simulink model "Torque_regulation_1_0"  (R2022b)
settings: Solver=VariableStepAuto  StartTime=0.0  StopTime=30  RelTol=1e-3
libraries: simulink x4, slpidlib x1
settings Model: Creator=tiszu  LastModifiedBy=tiszu

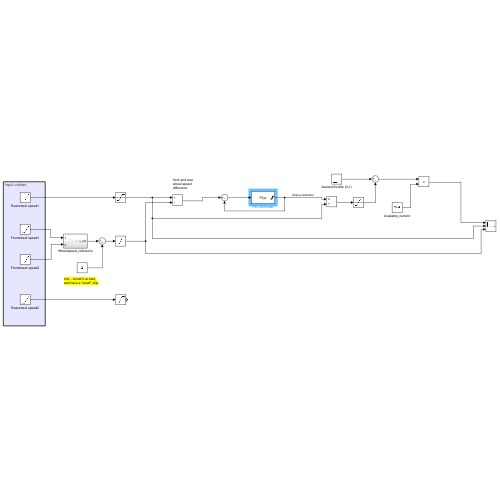
[thumbnail: Simulink's stored preview of the top-level diagram]
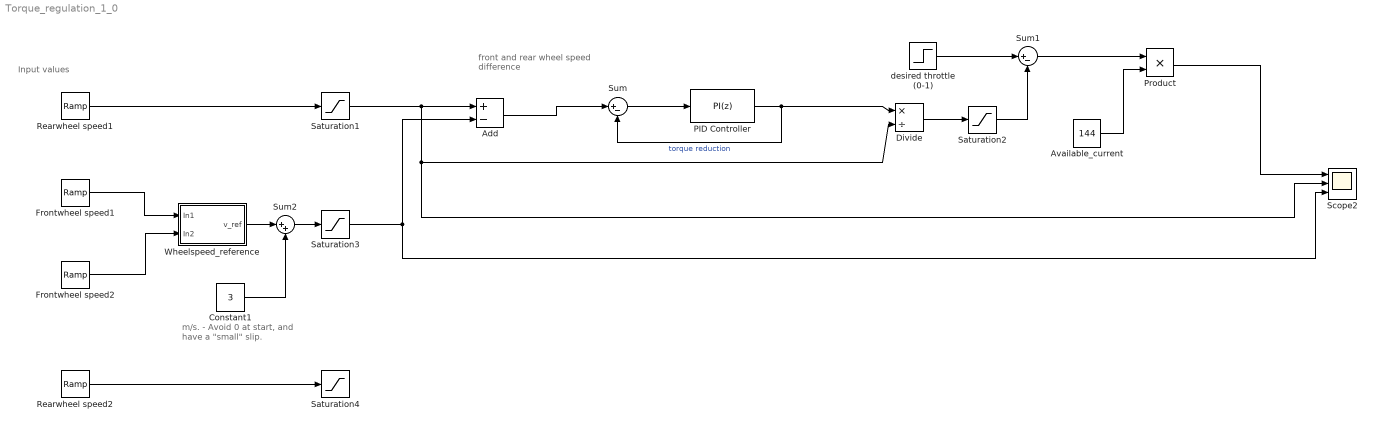
== system Torque_regulation_1_0 ==
  note: Input values
  note: m/s. - Avoid 0 at start, and have a "small" slip.
  note: front and rear wheel speed difference
  Add : Sum  Inputs=+-
  Available_current : Constant  Value=144
  Constant1 : Constant  Value=3
  Divide : Product  Inputs=*/
  Frontwheel speed1 : simulink/Sources/Ramp  slope=5  start=0  InitialOutput=0
  Frontwheel speed2 : simulink/Sources/Ramp  slope=5  start=0  InitialOutput=0
  PID Controller : slpidlib/PID Controller  Controller=PI  Form=Parallel  TimeDomain=Discrete-time  UseExternalTs=off  SampleTime=0.01  IntegratorMethod=Forward Euler  FilterMethod=Forward Euler  ControllerParametersSource=internal  P=0.01  I=2  UseKiTs=off  D=0  N=100  UseFilter=on  TunerSelectOption=Transfer Function Based (PID Tuner App)  InitialConditionSource=internal  InitialConditionForIntegrator=0  InitialConditionForFilter=0  DifferentiatorICPrevScaledInput=0  ExternalReset=none  TrackingMode=off  Kt=1  LimitOutput=on  SatLimitsSource=internal  UpperSaturationLimit=100  LowerSaturationLimit=0  LinearizeAsGain=on  AntiWindupMode=back-calculation  Kb=1  LimitIntegrator=off  UpperIntegratorSaturationLimit=inf  LowerIntegratorSaturationLimit=-inf  POutMin=[]  POutMax=[]  IOutMin=[]  IOutMax=[]  DOutMin=[]  DOutMax=[]  NOutMin=[]  NOutMax=[]  SumOutMin=[]  SumOutMax=[]  SaturationOutMin=[]  SaturationOutMax=[]  PParamMin=[]  PParamMax=[]  IParamMin=[]  IParamMax=[]  DParamMin=[]  DParamMax=[]  NParamMin=[]  NParamMax=[]  KbParamMin=[]  KbParamMax=[]  KtParamMin=[]  KtParamMax=[]  KbOutMin=[]  KbOutMax=[]  KtOutMin=[]  KtOutMax=[]  IntegratorOutMin=[]  IntegratorOutMax=[]  FilterOutMin=[]  FilterOutMax=[]  SumI1OutMin=[]  SumI1OutMax=[]  SumI2OutMin=[]  SumI2OutMax=[]  SumI3OutMin=[]  SumI3OutMax=[]  SumI4OutMin=[]  SumI4OutMax=[]  SumDOutMin=[]  SumDOutMax=[]  DifferentiatorOutMin=[]  DifferentiatorOutMax=[]  FilterDiffOutCoefMin=[]  FilterDiffOutCoefMax=[]  ReciprocalOutMin=[]  ReciprocalOutMax=[]  SumDenOutMin=[]  SumDenOutMax=[]  SumNumOutMin=[]  SumNumOutMax=[]  DivideOutMin=[]  DivideOutMax=[]  UdiffTsProdOutMin=[]  UdiffTsProdOutMax=[]  NTsProdOutMin=[]  NTsProdOutMax=[]  UintegralTsProdOutMin=[]  UintegralTsProdOutMax=[]  UngainTsProdOutMin=[]  UngainTsProdOutMax=[]  ClampingZeroOutDataTypeStr=Inherit: Inherit via back propagation  ClampingZeroOutMin=[]  ClampingZeroOutMax=[]  FilterDenConstantOutDataTypeStr=Inherit: Inherit via back propagation  FilterDenConstantOutMin=[]  FilterDenConstantOutMax=[]  PCopyOutDataTypeStr=Inherit: Inherit via back propagation  PCopyOutMin=[]  PCopyOutMax=[]  NCopyOutDataTypeStr=Inherit: Inherit via back propagation  NCopyOutMin=[]  NCopyOutMax=[]  IntegratorContinuousStateAttributes=''  IntegratorStateMustResolveToSignalObject=off  IntegratorRTWStateStorageClass=Auto  FilterContinuousStateAttributes=''  FilterStateMustResolveToSignalObject=off  FilterRTWStateStorageClass=Auto  ParallelPVariant=InternalParameters  IdealPVariant=Disabled  IVariant=InternalParameters  DVariant=Disabled  IntegratorVariant=Discrete  SatVariant=Enabled  AWVariant=BackCalculation  PCopyVariant=Disabled  TRVariant=Disabled  FdbkBlocksVariant=Forward  IdealPFdbkVariant=Disabled  SatFdbkVariant=Disabled  DerivativeFilterVariant=Disabled  NVariant=Disabled  NCopyVariant=Disabled_SignalSpec  FilterICVariant=Disabled  IntegratorICVariant=InternalICs  ExternalResetVariant=Disabled  TRSumVariant=Passthrough  SumFdbkVariant=Disabled  SumVariant=Sum_PI  TsampFilterVariant=InternalTs  TsampNgainVariant=Passthrough  TsampIntegralVariant=Passthrough  ExternalSaturationOutDataTypeStr=Inherit: Same as second input
  Product : Product
  Rearwheel speed1 : simulink/Sources/Ramp  slope=50  start=0  InitialOutput=0
  Rearwheel speed2 : simulink/Sources/Ramp  slope=100  start=0  InitialOutput=0
  Saturation1 : Saturate  UpperLimit=30  LowerLimit=0
  Saturation2 : Saturate  UpperLimit=1  LowerLimit=0
  Saturation3 : Saturate  UpperLimit=30  LowerLimit=0
  Saturation4 : Saturate  UpperLimit=100  LowerLimit=0
  Scope2 : Scope  NumInputPorts=3
  Sum : Sum  Inputs=|+-
  Sum1 : Sum  Inputs=|+-
  Sum2 : Sum  Inputs=|++
  Wheelspeed_reference : Subsystem
  desired throttle (0-1) : Step  Time=0  SampleTime=0
  wires:
  Available_current/1 -> Product/2
  Frontwheel speed1/1 -> Wheelspeed_reference/1(In1)
  Divide/1 -> Saturation2/1
  Sum1/1 -> Product/1
  Constant1/1 -> Sum2/2
  Frontwheel speed2/1 -> Wheelspeed_reference/2(In2)
  PID Controller/1 -> Sum/2, Divide/1  "torque reduction"
  Rearwheel speed2/1 -> Saturation4/1
  Saturation2/1 -> Sum1/2
  Wheelspeed_reference/1(v_ref) -> Sum2/1
  Rearwheel speed1/1 -> Saturation1/1
  Sum2/1 -> Saturation3/1
  Sum/1 -> PID Controller/1
  desired throttle (0-1)/1 -> Sum1/1
  Add/1 -> Sum/1
  Saturation1/1 -> Divide/2, Scope2/2, Add/1
  Product/1 -> Scope2/1
  Saturation3/1 -> Scope2/3, Add/2

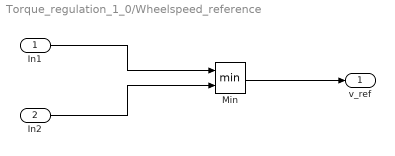
== system Torque_regulation_1_0/Wheelspeed_reference ==
  In1 : Inport
  In2 : Inport  Port=2
  Min : MinMax  Inputs=2
  v_ref : Outport
  wires:
  In1/1 -> Min/1
  Min/1 -> v_ref/1
  In2/1 -> Min/2
